simulink library "TranslationalDynamics3DoF"  (R2015a)
settings: Solver=ode45  StartTime=0.0  StopTime=10.0  RelTol=1e-3
undefined symbols (not defined in the file): Target
settings Model: Creator=bbrito  LastModifiedBy=bbrito

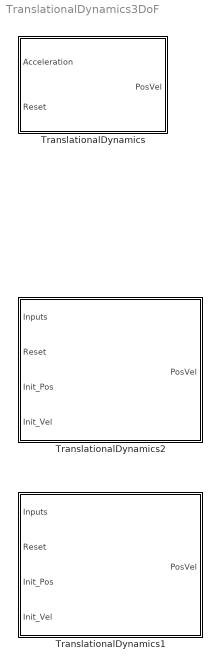
== system TranslationalDynamics3DoF ==
  TranslationalDynamics : Subsystem  TreatAsAtomicUnit=on  mask{v0=Target.ModelData.v0_CB, x0=Target.ModelData.x0_CB}
      mask prompts: v0 "Initial Velocity"; x0 "Initial Position"
  TranslationalDynamics1 : Subsystem  AncestorBlock=TranslationalDynamics3DoF/TranslationalDynamics2  TreatAsAtomicUnit=on
  TranslationalDynamics2 : Subsystem  AncestorBlock=TranslationalDynamics3DoF/TranslationalDynamics  TreatAsAtomicUnit=on

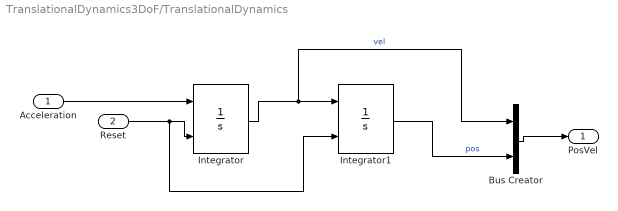
== system TranslationalDynamics3DoF/TranslationalDynamics ==
  Acceleration : Inport
  Reset : Inport  Port=2
  Bus Creator : BusCreator  Inputs=2
  Integrator : Integrator  ExternalReset=rising  InitialCondition=v0
  Integrator1 : Integrator  ExternalReset=rising  InitialCondition=x0
  PosVel : Outport
  wires:
  Reset/1 -> Integrator1/2, Integrator/2
  Bus Creator/1 -> PosVel/1
  Acceleration/1 -> Integrator/1
  Integrator/1 -> Integrator1/1, Bus Creator/1  "vel"
  Integrator1/1 -> Bus Creator/2  "pos"

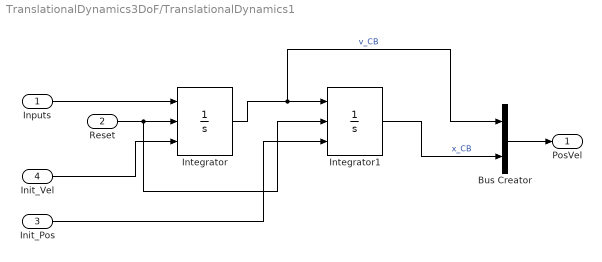
== system TranslationalDynamics3DoF/TranslationalDynamics1 ==
  Inputs : Inport
  Reset : Inport  Port=2
  Init_Pos : Inport  Port=3
  Init_Vel : Inport  Port=4
  Bus Creator : BusCreator  Inputs=2
  Integrator : Integrator  ExternalReset=rising  InitialConditionSource=external
  Integrator1 : Integrator  ExternalReset=rising  InitialConditionSource=external
  PosVel : Outport
  wires:
  Integrator1/1 -> Bus Creator/2  "x_CB"
  Integrator/1 -> Integrator1/1, Bus Creator/1  "v_CB"
  Inputs/1 -> Integrator/1
  Bus Creator/1 -> PosVel/1
  Reset/1 -> Integrator1/2, Integrator/2
  Init_Vel/1 -> Integrator/3
  Init_Pos/1 -> Integrator1/3

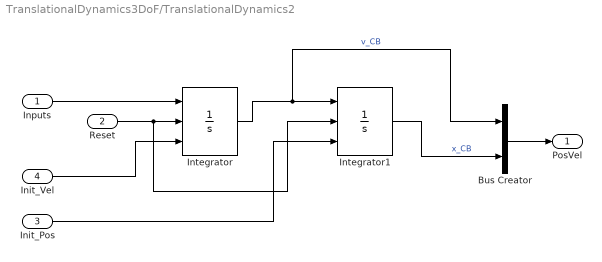
== system TranslationalDynamics3DoF/TranslationalDynamics2 ==
  Inputs : Inport
  Reset : Inport  Port=2
  Init_Pos : Inport  Port=3
  Init_Vel : Inport  Port=4
  Bus Creator : BusCreator  Inputs=2
  Integrator : Integrator  ExternalReset=rising  InitialConditionSource=external
  Integrator1 : Integrator  ExternalReset=rising  InitialConditionSource=external
  PosVel : Outport
  wires:
  Integrator1/1 -> Bus Creator/2  "x_CB"
  Integrator/1 -> Integrator1/1, Bus Creator/1  "v_CB"
  Inputs/1 -> Integrator/1
  Bus Creator/1 -> PosVel/1
  Reset/1 -> Integrator1/2, Integrator/2
  Init_Vel/1 -> Integrator/3
  Init_Pos/1 -> Integrator1/3
